simulink model "powerwindow_ec"  (R2019a)
settings: Solver=FixedStepDiscrete  StartTime=0.0  StopTime=20.0  FixedStep=0.01  RelTol=1e-3
values from neighbouring files (symbols this model uses):
  auto_down_time = copy(auto_up_time)    [powerwindow_ec_init.m]
  auto_up_time = Simulink.Parameter    [powerwindow_ec_init.m]
  bFALSE = Simulink.Parameter    [powerwindow_ec_init.m]
  emergency_down_time = copy(auto_up_time)    [powerwindow_ec_init.m]
  position_endstop_top = Simulink.Parameter    [powerwindow_ec_init.m]
settings Model: TunableVars=auto_down_time,auto_up_time,emergency_down_time,position_endstop_top  TunableVarsStorageClass=Auto,Auto,Auto,Auto  TunableVarsTypeQualifier=,,,  Creator=Wolfgang Meincke  LastModifiedBy=yatishc
settings DataIOCC: LimitDataPoints=on  SaveFormat=Array  ReturnWorkspaceOutputs=off
settings OptimizationCC: BlockReduction=off  BooleanDataType=off  ConditionallyExecuteInputs=off  DefaultParameterBehavior=Inlined  GlobalBufferReuse=off  EnableMemcpy=off  ExpressionDepthLimit=2147483647  ZeroExternalMemoryAtStartup=off  ZeroInternalMemoryAtStartup=off  InitFltsAndDblsToZero=on  NoFixptDivByZeroProtection=on  LifeSpan=1
settings DebuggingCC: RTPrefix=none  SaveWithParameterizedLinksMsg=none  UnderspecifiedInitializationDetection=Classic  MergeDetectMultiDrivingBlocksExec=none  MultiTaskDSMMsg=warning  MultiTaskCondExecSysMsg=none  ParameterPrecisionLossMsg=none  FcnCallInpInsideContextMsg=warning  UnconnectedInputMsg=none  UnconnectedOutputMsg=none  AllowSymbolicDim=off  StateNameClashWarn=warning  SFUnexpectedBacktrackingDiag=warning  SFNoUnconditionalDefaultTransitionDiag=warning  SFExecutionAtInitializationDiag=none  ArithmeticOperatorsInVariantConditions=warning
settings HardwareCC: ProdLongLongMode=on
settings ModelReferenceCC: ModelReferenceNumInstancesAllowed=Single  PropagateSignalLabelsOutOfModel=off
settings SFSimCC: SimUseLocalCustomCode=off  SimParseCustomCode=off  MATLABDynamicMemAlloc=off
settings RTWCC: SystemTargetFile=ert.tlc  GenCodeOnly=on  TemplateMakefile=ert_default_tmf  RetainRTWFile=on  RTWUseLocalCustomCode=off  Toolchain=LCC-win64 v2.4.1 | gmake (64-bit Windows)  PortableWordSizes=on
settings CodeAppCC: IgnoreCustomStorageClasses=off  MaxIdLength=40  StateflowObjectComments=on
settings ERTTargetCC: MultiwordLength=2048  IncludeMdlTerminateFcn=off  CombineSignalStateStructs=on  SupportAbsoluteTime=off  LogVarNameModifier=_rt  PurelyIntegerCode=on  SupportNonFinite=off  SupportComplex=off  RemoveResetFunc=off  RootIOFormat=Part of model data structure  ERTCustomFileTemplate=example_file_process.tlc  ConvertIfToSwitch=off  SuppressUnreachableDefaultCases=off
settings ConfigComp: CovMetricSettings=dw  CovSaveCumulativeToWorkspaceVar=on  CovSaveSingleToWorkspaceVar=on  CovExternalEMLEnable=off  CovSFcnEnable=off

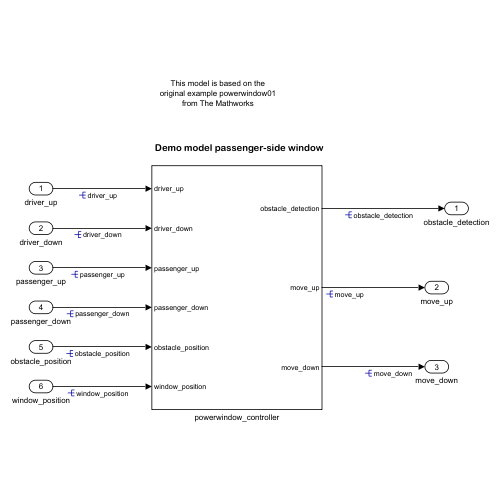
[thumbnail: Simulink's stored preview of the top-level diagram]
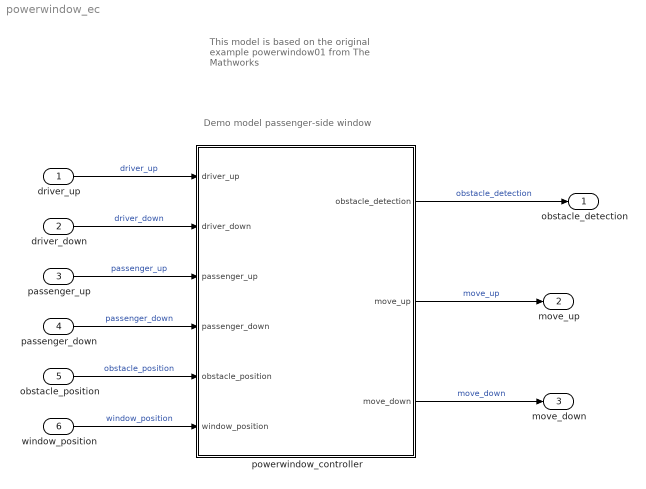
== system powerwindow_ec ==
  note: This model is based on the
      | original example powerwindow01
      | from The Mathworks
  note: Demo model passenger-side window
  driver_up : Inport  OutMin=0  OutMax=1
  driver_down : Inport  Port=2  OutMin=0  OutMax=1
  passenger_up : Inport  Port=3  OutMin=0  OutMax=1
  passenger_down : Inport  Port=4  OutMin=0  OutMax=1
  obstacle_position : Inport  Port=5  OutMin=0  OutMax=0.45  OutDataTypeStr=fixdt(0,16,0.001,0)
  window_position : Inport  Port=6  OutMin=0  OutMax=0.45  OutDataTypeStr=fixdt(0,16,0.001,0)
  powerwindow_controller : Subsystem  RTWFcnName=powerwindow_controller
      settings: RTWSystemCode=Nonreusable function  RTWFcnNameOpts=User specified  RTWFileNameOpts=Use function name
  obstacle_detection : Outport  OutMin=0  OutMax=1  VectorParamsAs1DForOutWhenUnconnected=off
  move_up : Outport  Port=2  OutMin=0  OutMax=1  VectorParamsAs1DForOutWhenUnconnected=off
  move_down : Outport  Port=3  OutMin=0  OutMax=1  VectorParamsAs1DForOutWhenUnconnected=off
  wires:
  driver_up/1 -> powerwindow_controller/1(driver_up)  "driver_up"
  driver_down/1 -> powerwindow_controller/2(driver_down)  "driver_down"
  passenger_up/1 -> powerwindow_controller/3(passenger_up)  "passenger_up"
  passenger_down/1 -> powerwindow_controller/4(passenger_down)  "passenger_down"
  obstacle_position/1 -> powerwindow_controller/5(obstacle_position)  "obstacle_position"
  window_position/1 -> powerwindow_controller/6(window_position)  "window_position"
  powerwindow_controller/1(obstacle_detection) -> obstacle_detection/1  "obstacle_detection"
  powerwindow_controller/2(move_up) -> move_up/1  "move_up"
  powerwindow_controller/3(move_down) -> move_down/1  "move_down"

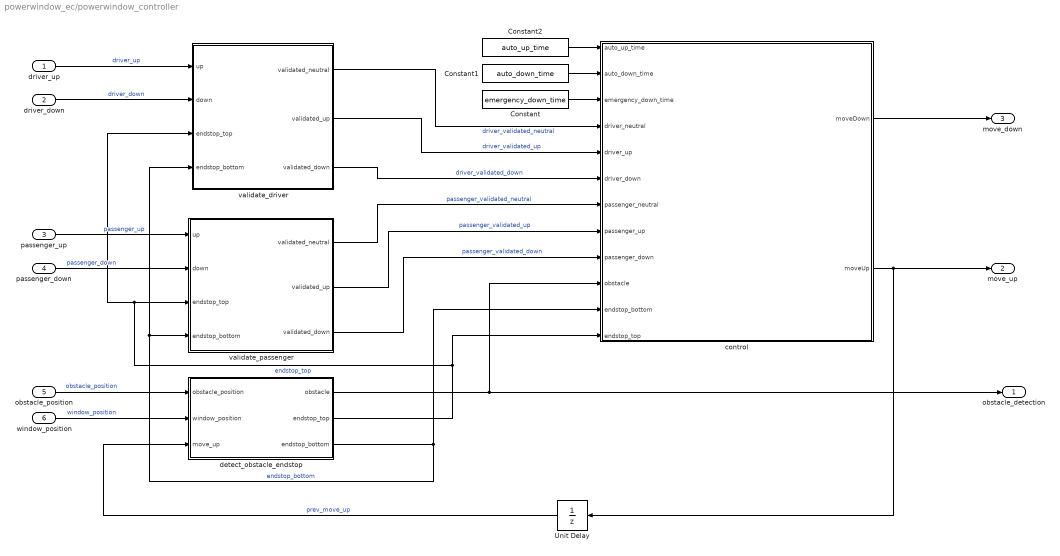
== system powerwindow_ec/powerwindow_controller ==
  driver_up : Inport  RequirementInfo={} %GIDa_c35cf34b_45f5_487d_8434_6977e2d5d2f3  OutMin=0  OutMax=1  OutDataTypeStr=boolean  PortDimensions=1
  driver_down : Inport  RequirementInfo={} %GIDa_825829a4_4c67_4036_abe4_d775b7ffbdb6  Port=2  OutMin=0  OutMax=1  OutDataTypeStr=boolean
  passenger_up : Inport  RequirementInfo={} %GIDa_896a61d0_51a5_427e_b548_01888eb9493f  Port=3  OutMin=0  OutMax=1  OutDataTypeStr=boolean  PortDimensions=1
  passenger_down : Inport  RequirementInfo={} %GIDa_acad868a_9832_4517_80f1_eb2c424aca82  Port=4  OutMin=0  OutMax=1  OutDataTypeStr=boolean  PortDimensions=1
  obstacle_position : Inport  RequirementInfo={} %GIDa_5be180b3_640c_44df_b132_7c12c9dd4782  Port=5  OutMin=0  OutMax=0.45  OutDataTypeStr=fixdt(0,16,0.001,0)  PortDimensions=1
  window_position : Inport  RequirementInfo={} %GIDa_279514cf_fecf_4861_97d0_86738c273b33  Port=6  OutMin=0  OutMax=0.45  OutDataTypeStr=fixdt(0,16,0.001,0)  PortDimensions=1
  Constant : Constant  RequirementInfo={} %GIDa_9514aab4_7290_4656_a952_a9cac9bec120  Value=emergency_down_time  OutMin=0  OutMax=255  OutDataTypeStr=uint8
  Constant1 : Constant  RequirementInfo={} %GIDa_6c74b792_e839_4a12_ac84_86c7d570a533  Value=auto_down_time  OutMin=0  OutMax=255  OutDataTypeStr=uint8
  Constant2 : Constant  RequirementInfo={} %GIDa_27bbea0c_c5f9_4e52_b093_a1cd3ec1797f  Value=auto_up_time  OutMin=0  OutMax=255  OutDataTypeStr=uint8
  Unit Delay : UnitDelay  RequirementInfo={} %GIDa_61c3f994_badd_4b85_b577_84166d45c76a  SampleTime=-1  HasFrameUpgradeWarning=on
  control : Stateflow chart  RequirementInfo={} %GIDa_03dc6751_b1fa_4801_9ce5_d6a4ecb5c081
      settings: FunctionInterfaceSpec=Allow arguments
  detect_obstacle_endstop : Subsystem  Description=""  TreatAsAtomicUnit=on  RTWFcnName=detect_obstacle_endstop
      settings: AttributesFormatString=%<Description>  RTWSystemCode=Nonreusable function  RTWFcnNameOpts=User specified  RTWFileNameOpts=Use subsystem name
  validate_driver : Subsystem  TreatAsAtomicUnit=on  RTWFcnName=validate_driver
      settings: RTWSystemCode=Nonreusable function  RTWFcnNameOpts=User specified  RTWFileNameOpts=Use subsystem name
  validate_passenger : Subsystem  RequirementInfo={} %GIDa_33b218b3_9db5_4fe6_9638_6b05429d8e58  TreatAsAtomicUnit=on  RTWFcnName=validate_passenger
      settings: RTWSystemCode=Nonreusable function  RTWFcnNameOpts=User specified  RTWFileNameOpts=Use function name
  obstacle_detection : Outport  RequirementInfo={} %GIDa_4eefd6fd_6a0d_4232_ac82_ccb47f3c36e3  OutMin=0  OutMax=1  OutDataTypeStr=boolean  PortDimensions=1  VectorParamsAs1DForOutWhenUnconnected=off
  move_up : Outport  RequirementInfo={} %GIDa_cfaa6890_1b09_43c8_9181_c9775bd2e746  Port=2  OutMin=0  OutMax=1  OutDataTypeStr=boolean  PortDimensions=1  VectorParamsAs1DForOutWhenUnconnected=off
  move_down : Outport  RequirementInfo={} %GIDa_e72b7e0a_8232_4793_901f_580fad4f0530  Port=3  OutMin=0  OutMax=1  OutDataTypeStr=boolean  PortDimensions=1  VectorParamsAs1DForOutWhenUnconnected=off
  wires:
  detect_obstacle_endstop/3(endstop_bottom) -> validate_driver/4(endstop_bottom), validate_passenger/4(endstop_bottom), control/11(endstop_bottom)  "endstop_bottom"
  detect_obstacle_endstop/2(endstop_top) -> control/12(endstop_top), validate_driver/3(endstop_top), validate_passenger/3(endstop_top)  "endstop_top"
  validate_passenger/3(validated_down) -> control/9(passenger_down)  "passenger_validated_down"
  validate_passenger/2(validated_up) -> control/8(passenger_up)  "passenger_validated_up"
  validate_passenger/1(validated_neutral) -> control/7(passenger_neutral)  "passenger_validated_neutral"
  validate_driver/3(validated_down) -> control/6(driver_down)  "driver_validated_down"
  validate_driver/2(validated_up) -> control/5(driver_up)  "driver_validated_up"
  validate_driver/1(validated_neutral) -> control/4(driver_neutral)  "driver_validated_neutral"
  Constant/1 -> control/3(emergency_down_time)
  Constant1/1 -> control/2(auto_down_time)
  Constant2/1 -> control/1(auto_up_time)
  control/1(moveDown) -> move_down/1
  control/2(moveUp) -> move_up/1, Unit Delay/1
  detect_obstacle_endstop/1(obstacle) -> control/10(obstacle), obstacle_detection/1
  Unit Delay/1 -> detect_obstacle_endstop/3(move_up)  "prev_move_up"
  window_position/1 -> detect_obstacle_endstop/2(window_position)  "window_position"
  obstacle_position/1 -> detect_obstacle_endstop/1(obstacle_position)  "obstacle_position"
  passenger_down/1 -> validate_passenger/2(down)  "passenger_down"
  passenger_up/1 -> validate_passenger/1(up)  "passenger_up"
  driver_down/1 -> validate_driver/2(down)  "driver_down"
  driver_up/1 -> validate_driver/1(up)  "driver_up"

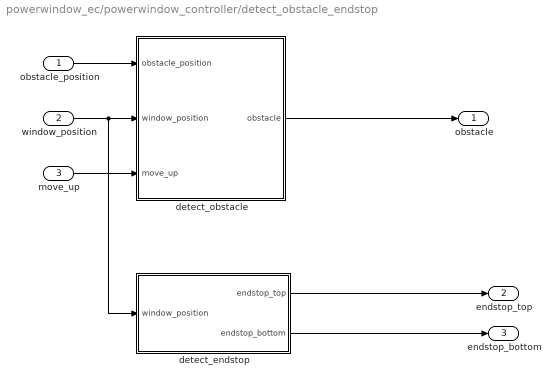
== system powerwindow_ec/powerwindow_controller/detect_obstacle_endstop ==
  obstacle_position : Inport  RequirementInfo={} %GIDa_2c523ff6_7978_4731_916d_ba96442347ee
  window_position : Inport  RequirementInfo={} %GIDa_e1d20317_e3ef_4a09_9a0f_4281293c9f26  Port=2
  move_up : Inport  RequirementInfo={} %GIDa_5f38f6b1_95fb_4aef_ba44_8aaabe685aa5  Port=3
  detect_endstop : Subsystem  RequirementInfo={} %GIDa_2593335f_ebb0_43cf_9a39_2217339a862c
  detect_obstacle : Subsystem  RequirementInfo={} %GIDa_68f09a5d_865e_4d80_9553_6123df56ce2c
  obstacle : Outport  RequirementInfo={} %GIDa_76b93d49_6133_4f74_9957_e79afe91ce74  VectorParamsAs1DForOutWhenUnconnected=off
  endstop_top : Outport  RequirementInfo={} %GIDa_88a654a8_9697_4d16_b6ed_e9fe94316691  Port=2  VectorParamsAs1DForOutWhenUnconnected=off
  endstop_bottom : Outport  RequirementInfo={} %GIDa_79e1bc3d_40d8_4ea1_ab03_899f1380a234  Port=3  VectorParamsAs1DForOutWhenUnconnected=off
  wires:
  detect_endstop/2(endstop_bottom) -> endstop_bottom/1
  detect_endstop/1(endstop_top) -> endstop_top/1
  detect_obstacle/1(obstacle) -> obstacle/1
  obstacle_position/1 -> detect_obstacle/1(obstacle_position)
  window_position/1 -> detect_endstop/1(window_position), detect_obstacle/2(window_position)
  move_up/1 -> detect_obstacle/3(move_up)

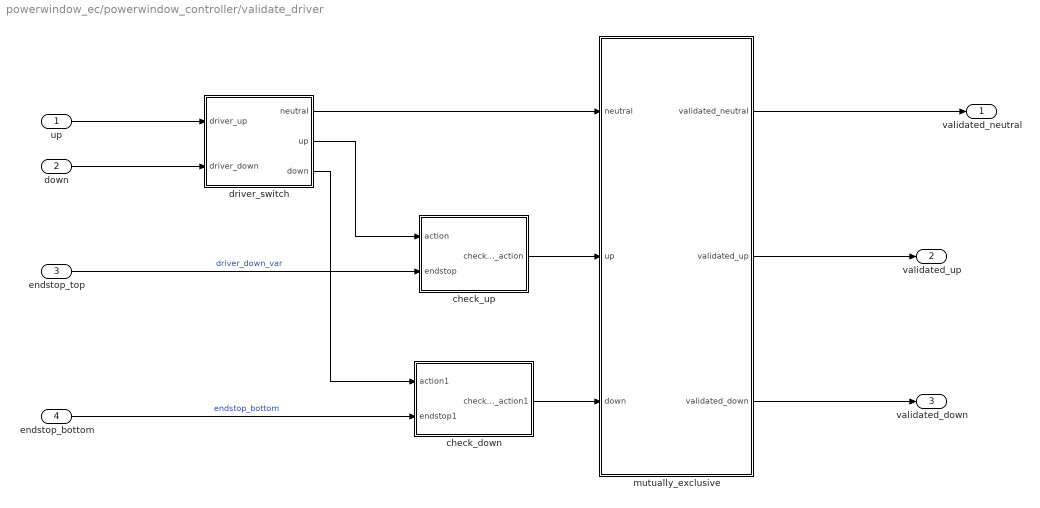
== system powerwindow_ec/powerwindow_controller/validate_driver ==
  up : Inport  RequirementInfo={} %GIDa_0f060a46_f46d_4ca9_9fdd_5b4ef64425ee  OutDataTypeStr=boolean  PortDimensions=1  SampleTime=[0.01,0]
  down : Inport  RequirementInfo={} %GIDa_ee71ce1a_69e4_43ae_938d_beeecc753a79  Port=2  OutDataTypeStr=boolean  PortDimensions=1  SampleTime=[0.01,0]
  endstop_top : Inport  RequirementInfo={} %GIDa_950bdb33_ed63_463b_ae82_db42f04fc79f  Port=3  OutDataTypeStr=boolean  PortDimensions=1  SampleTime=[0.01,0]
  endstop_bottom : Inport  RequirementInfo={} %GIDa_82fa3d1b_deb6_4fcf_98df_c73a1f0760dd  Port=4  OutDataTypeStr=boolean  PortDimensions=1  SampleTime=[0.01,0]
  check_down : Subsystem  RequirementInfo={} %GIDa_88cdc8aa_9e17_4d6d_82ad_f4b053a158b5
  check_up : Subsystem  RequirementInfo={} %GIDa_f004a38e_b1e3_4775_9b61_543b39059229
  driver_switch : Subsystem  RequirementInfo={} %GIDa_0ddca807_3145_43f8_91cf_ba07f3905be6
  mutually_exclusive : Subsystem  RequirementInfo={} %GIDa_48603077_07ff_4607_938a_0c2458af8a7a
  validated_neutral : Outport  RequirementInfo={} %GIDa_93510d49_6043_4ebc_8207_b7ce98567d3f  OutDataTypeStr=boolean  PortDimensions=1  SampleTime=[0.01,0]  VectorParamsAs1DForOutWhenUnconnected=off
  validated_up : Outport  RequirementInfo={} %GIDa_e717bde8_9582_4b32_98f4_cb8fdf2291d3  Port=2  OutDataTypeStr=boolean  PortDimensions=1  SampleTime=[0.01,0]  VectorParamsAs1DForOutWhenUnconnected=off
  validated_down : Outport  RequirementInfo={} %GIDa_99f1727e_ebb0_4d17_9343_1d6808b3939a  Port=3  OutDataTypeStr=boolean  PortDimensions=1  SampleTime=[0.01,0]  VectorParamsAs1DForOutWhenUnconnected=off
  wires:
  mutually_exclusive/3(validated_down) -> validated_down/1
  mutually_exclusive/2(validated_up) -> validated_up/1
  mutually_exclusive/1(validated_neutral) -> validated_neutral/1
  check_down/1(checked_action1) -> mutually_exclusive/3(down)
  check_up/1(checked_action) -> mutually_exclusive/2(up)
  driver_switch/1(neutral) -> mutually_exclusive/1(neutral)
  endstop_bottom/1 -> check_down/2(endstop1)  "endstop_bottom"
  endstop_top/1 -> check_up/2(endstop)  "driver_down_var"
  driver_switch/3(down) -> check_down/1(action1)
  driver_switch/2(up) -> check_up/1(action)
  down/1 -> driver_switch/2(driver_down)
  up/1 -> driver_switch/1(driver_up)

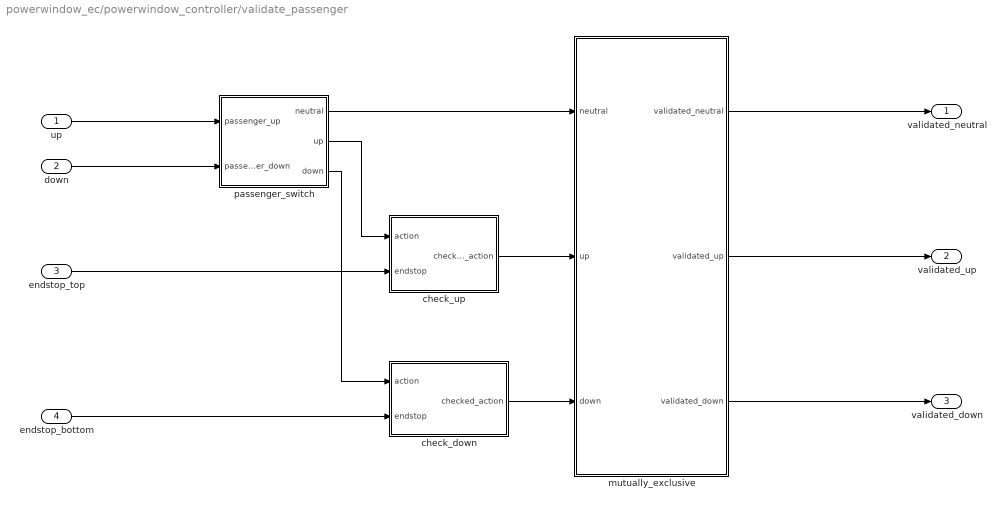
== system powerwindow_ec/powerwindow_controller/validate_passenger ==
  up : Inport  RequirementInfo={} %GIDa_b6408152_b334_4925_a16c_3622ca90ad97
  down : Inport  RequirementInfo={} %GIDa_df58e8e8_afe3_46fe_9c17_76802ca163b9  Port=2
  endstop_top : Inport  RequirementInfo={} %GIDa_230b0d07_e7b6_4a10_b2ed_43443fa38605  Port=3
  endstop_bottom : Inport  RequirementInfo={} %GIDa_91eacfdf_7e8f_4c54_b206_f15636a3f59e  Port=4
  check_down : Subsystem  RequirementInfo={} %GIDa_62b405b0_f053_4287_a6d2_c18d3e3b6c5b
  check_up : Subsystem  RequirementInfo={} %GIDa_92e78854_fa4d_4c59_81d3_3ea0d0c4a8a4
  mutually_exclusive : Subsystem  RequirementInfo={} %GIDa_5d841e18_2fc4_47d2_8782_e39db535edd2
  passenger_switch : Subsystem  RequirementInfo={} %GIDa_1746543f_6789_44d7_a576_254e44230f82
  validated_neutral : Outport  RequirementInfo={} %GIDa_ebd107f4_f924_4fcc_86d4_5bdc2b7613d2  VectorParamsAs1DForOutWhenUnconnected=off
  validated_up : Outport  RequirementInfo={} %GIDa_a655668a_fb1a_4125_a470_9ec06e9de417  Port=2  VectorParamsAs1DForOutWhenUnconnected=off
  validated_down : Outport  RequirementInfo={} %GIDa_d891aac2_9896_4b15_add3_213d9f963ba8  Port=3  VectorParamsAs1DForOutWhenUnconnected=off
  wires:
  check_down/1(checked_action) -> mutually_exclusive/3(down)
  check_up/1(checked_action) -> mutually_exclusive/2(up)
  passenger_switch/1(neutral) -> mutually_exclusive/1(neutral)
  endstop_bottom/1 -> check_down/2(endstop)
  endstop_top/1 -> check_up/2(endstop)
  passenger_switch/3(down) -> check_down/1(action)
  passenger_switch/2(up) -> check_up/1(action)
  down/1 -> passenger_switch/2(passenger_down)
  up/1 -> passenger_switch/1(passenger_up)
  mutually_exclusive/1(validated_neutral) -> validated_neutral/1
  mutually_exclusive/2(validated_up) -> validated_up/1
  mutually_exclusive/3(validated_down) -> validated_down/1

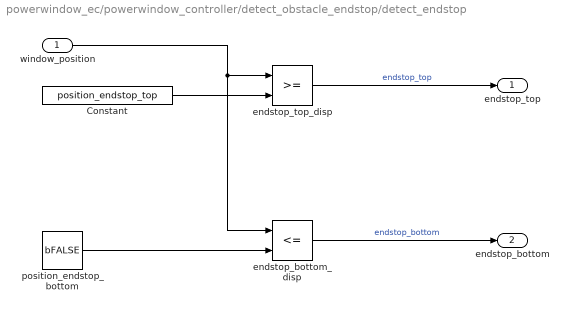
== system powerwindow_ec/powerwindow_controller/detect_obstacle_endstop/detect_endstop ==
  window_position : Inport  RequirementInfo={} %GIDa_5272641f_60a5_49ab_860f_474d665ad38c
  Constant : Constant  RequirementInfo={} %GIDa_b00b9cbe_3e72_4b2c_8740_e9f730c36594  Value=position_endstop_top  OutMin=0.35  OutMax=0.45  OutDataTypeStr=fixdt(0,16,0.001,0)
  endstop_bottom_disp : RelationalOperator  RequirementInfo={} %GIDa_d55d2907_c327_453e_a02b_45678f8411a7  Operator=<=  OutDataTypeStr=boolean  RndMeth=Nearest
      settings: AttributesFormatString=%<Description>
  endstop_top_disp : RelationalOperator  RequirementInfo={} %GIDa_6f4ae952_2810_4851_a41e_34cbed529beb  OutDataTypeStr=boolean  RndMeth=Nearest
      settings: AttributesFormatString=%<Description>
  position_endstop_bottom : Constant  RequirementInfo={} %GIDa_07897626_90bb_46f7_9dcd_03d3ee392bc4  Value=bFALSE  OutDataTypeStr=Inherit: Inherit via back propagation
  endstop_top : Outport  RequirementInfo={} %GIDa_6bdb3a67_ce18_47c7_a161_80224aafb80a  VectorParamsAs1DForOutWhenUnconnected=off
  endstop_bottom : Outport  RequirementInfo={} %GIDa_4cae9334_ebd9_4f06_b7b7_b5123c42f3a3  Port=2  VectorParamsAs1DForOutWhenUnconnected=off
  wires:
  endstop_bottom_disp/1 -> endstop_bottom/1  "endstop_bottom"
  endstop_top_disp/1 -> endstop_top/1  "endstop_top"
  position_endstop_bottom/1 -> endstop_bottom_disp/2
  window_position/1 -> endstop_bottom_disp/1, endstop_top_disp/1
  Constant/1 -> endstop_top_disp/2

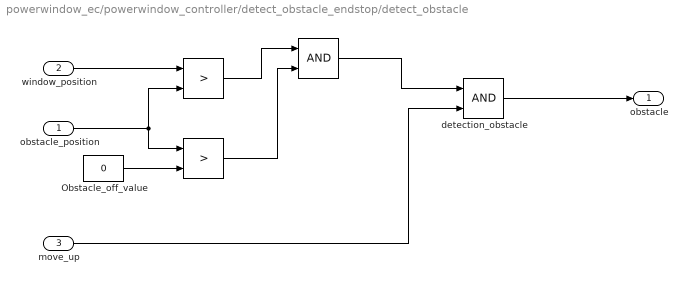
== system powerwindow_ec/powerwindow_controller/detect_obstacle_endstop/detect_obstacle ==
  obstacle_position : Inport  RequirementInfo={} %GIDa_f04cc014_84fe_4f3b_ba9a_4eb089b94b63
  window_position : Inport  RequirementInfo={} %GIDa_6efc2069_33c6_4baf_bb03_5d2172fe3169  Port=2
  move_up : Inport  RequirementInfo={} %GIDa_bfb3c774_9ca6_457c_ba9e_d7bb12997122  Port=3
  " " : Logic  RequirementInfo={} %GIDa_42f9d249_5a3b_49ec_af0d_2273563bb9a1  AllPortsSameDT=off  OutDataTypeStr=boolean
  "  " : RelationalOperator  RequirementInfo={} %GIDa_343b1761_e03d_4050_a63c_743fa9e53550  Operator=>  OutDataTypeStr=boolean  RndMeth=Nearest
  "   " : RelationalOperator  RequirementInfo={} %GIDa_d6c6c9bb_2e51_4c9f_94b3_dde6a683bc5b  Operator=>  OutDataTypeStr=boolean  RndMeth=Nearest
  Obstacle_off_value : Constant  RequirementInfo={} %GIDa_540ff0bd_b260_4aef_ac1e_5afd8b8de081  Value=0  OutDataTypeStr=Inherit: Inherit via back propagation
  detection_obstacle : Logic  RequirementInfo={} %GIDa_5a6fd671_9493_4039_aef6_1fac1883fec8  AllPortsSameDT=off  OutDataTypeStr=boolean
      settings: AttributesFormatString=%<Description>
  obstacle : Outport  RequirementInfo={} %GIDa_ab82724c_4453_4aa5_ac53_ecd73d5c0fd6  VectorParamsAs1DForOutWhenUnconnected=off
  wires:
  Obstacle_off_value/1 -> "   "/2
  obstacle_position/1 -> "  "/2, "   "/1
  "   "/1 -> " "/2
  move_up/1 -> detection_obstacle/2
  " "/1 -> detection_obstacle/1
  "  "/1 -> " "/1
  window_position/1 -> "  "/1
  detection_obstacle/1 -> obstacle/1

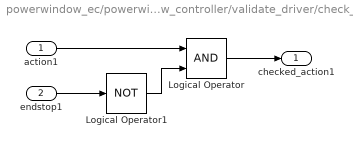
== system powerwindow_ec/powerwindow_controller/validate_driver/check_down ==
  action1 : Inport  RequirementInfo={} %GIDa_3bea607a_e8f1_4bd2_a5f0_c2e6970bbc31
  endstop1 : Inport  RequirementInfo={} %GIDa_b30aff22_abef_418a_aed3_192febbd33c5  Port=2
  Logical Operator : Logic  AllPortsSameDT=off  OutDataTypeStr=boolean
  Logical Operator1 : Logic  Operator=NOT  Inputs=1  AllPortsSameDT=off  OutDataTypeStr=boolean
  checked_action1 : Outport  RequirementInfo={} %GIDa_8daec588_ef56_4936_8f9d_ed4af0951a10  VectorParamsAs1DForOutWhenUnconnected=off
  wires:
  endstop1/1 -> Logical Operator1/1
  Logical Operator/1 -> checked_action1/1
  Logical Operator1/1 -> Logical Operator/2
  action1/1 -> Logical Operator/1

== system powerwindow_ec/powerwindow_controller/validate_driver/check_up ==
  action : Inport  RequirementInfo={} %GIDa_9887e9dd_28c6_4b8e_b0fa_e095af16b520
  endstop : Inport  RequirementInfo={} %GIDa_79f905fe_3050_4c1a_8e5e_85f3f37208eb  Port=2
  allow_action : Logic  RequirementInfo={} %GIDa_09215300_f454_41b9_9b13_3a6b54dcdb01  AllPortsSameDT=off  OutDataTypeStr=boolean
  not : Logic  RequirementInfo={} %GIDa_be8a7272_98c5_4194_9012_a918274462da  Operator=NOT  Inputs=1  AllPortsSameDT=off  OutDataTypeStr=boolean
  checked_action : Outport  RequirementInfo={} %GIDa_b7f1b7cb_7832_4f29_af81_202507dbc915  VectorParamsAs1DForOutWhenUnconnected=off
  wires:
  allow_action/1 -> checked_action/1  "checked_action"
  action/1 -> allow_action/1
  endstop/1 -> not/1
  not/1 -> allow_action/2

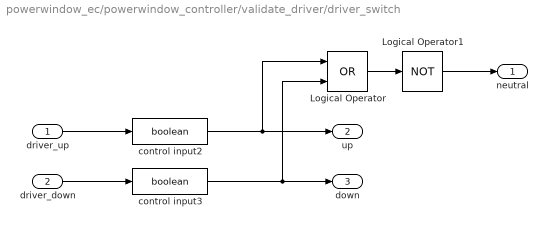
== system powerwindow_ec/powerwindow_controller/validate_driver/driver_switch ==
  driver_up : Inport  RequirementInfo={} %GIDa_b53eff7b_7dc7_4b26_a194_aca0440f3996
  driver_down : Inport  RequirementInfo={} %GIDa_850956fa_c58b_4722_af1c_699108fc9784  Port=2
  Logical Operator : Logic  RequirementInfo={} %GIDa_8ae19579_a7a5_4eb8_a8aa_b68c217ba182  Operator=OR  AllPortsSameDT=off  OutDataTypeStr=boolean
  Logical Operator1 : Logic  RequirementInfo={} %GIDa_e8e7857d_ce8d_43ef_928a_5ed594e12653  Operator=NOT  Inputs=1  AllPortsSameDT=off  OutDataTypeStr=boolean
  control input2 : DataTypeConversion  RequirementInfo={} %GIDa_c304843a_b249_46a1_bea1_8ad250524def  OutDataTypeStr=boolean  SaturateOnIntegerOverflow=on  RndMeth=Zero
  control input3 : DataTypeConversion  RequirementInfo={} %GIDa_1c10a33f_0b47_4b11_a97c_aa2c91a9423b  OutDataTypeStr=boolean  SaturateOnIntegerOverflow=on  RndMeth=Zero
  neutral : Outport  RequirementInfo={} %GIDa_6e66f8dd_3723_444f_a5c4_c8719978f12f  VectorParamsAs1DForOutWhenUnconnected=off
  up : Outport  RequirementInfo={} %GIDa_05276151_0839_48b1_ac06_cf6d99189f1e  Port=2  VectorParamsAs1DForOutWhenUnconnected=off
  down : Outport  RequirementInfo={} %GIDa_0ba51152_1781_4604_a294_81c93cdb2e1b  Port=3  VectorParamsAs1DForOutWhenUnconnected=off
  wires:
  driver_up/1 -> control input2/1
  driver_down/1 -> control input3/1
  control input2/1 -> up/1, Logical Operator/1
  control input3/1 -> down/1, Logical Operator/2
  Logical Operator/1 -> Logical Operator1/1
  Logical Operator1/1 -> neutral/1

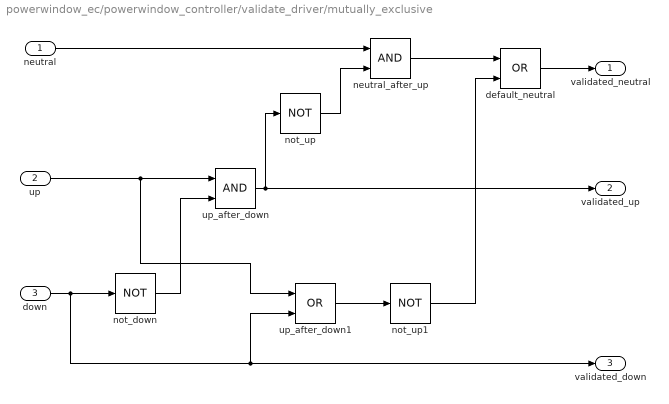
== system powerwindow_ec/powerwindow_controller/validate_driver/mutually_exclusive ==
  neutral : Inport  RequirementInfo={} %GIDa_02afa0c6_3e9f_4860_8ea3_38f0b34e8af7
  up : Inport  RequirementInfo={} %GIDa_1ebb9c89_44c5_40ac_900f_75ef026c92ad  Port=2
  down : Inport  RequirementInfo={} %GIDa_ad4b4981_c47d_4d30_8d96_b337e2a28fab  Port=3
  default_neutral : Logic  RequirementInfo={} %GIDa_68c2c660_39d6_4c62_9a3a_19199413336b  Operator=OR  AllPortsSameDT=off  OutDataTypeStr=boolean
  neutral_after_up : Logic  RequirementInfo={} %GIDa_7e258c9e_2c01_4723_a13f_4f5e92480034  AllPortsSameDT=off  OutDataTypeStr=boolean
  not_down : Logic  RequirementInfo={} %GIDa_a256d950_ec2d_4e87_a052_2312a72abf35  Operator=NOT  Inputs=1  AllPortsSameDT=off  OutDataTypeStr=boolean
  not_up : Logic  RequirementInfo={} %GIDa_f2e45f11_593e_44a0_9f62_a4dedafdeaaa  Operator=NOT  Inputs=1  AllPortsSameDT=off  OutDataTypeStr=boolean
  not_up1 : Logic  RequirementInfo={} %GIDa_57241b58_9572_4fb8_96d3_b88159c194b1  Operator=NOT  Inputs=1  AllPortsSameDT=off  OutDataTypeStr=boolean
  up_after_down : Logic  RequirementInfo={} %GIDa_f2858def_6366_414f_b896_53e3e935ca29  AllPortsSameDT=off  OutDataTypeStr=boolean
  up_after_down1 : Logic  RequirementInfo={} %GIDa_c5cf92de_e71e_48a0_b3a2_b9222e289e08  Operator=OR  AllPortsSameDT=off  OutDataTypeStr=boolean
  validated_neutral : Outport  RequirementInfo={} %GIDa_5fe76ab9_064b_4710_a12f_97d13d073964  VectorParamsAs1DForOutWhenUnconnected=off
  validated_up : Outport  RequirementInfo={} %GIDa_2868f914_1275_4356_93d2_c378fc22247d  Port=2  VectorParamsAs1DForOutWhenUnconnected=off
  validated_down : Outport  RequirementInfo={} %GIDa_b1de4b41_5c80_4a3b_8187_9415b836eb74  Port=3  VectorParamsAs1DForOutWhenUnconnected=off
  wires:
  neutral/1 -> neutral_after_up/1
  not_up/1 -> neutral_after_up/2
  up_after_down/1 -> validated_up/1, not_up/1
  up/1 -> up_after_down/1, up_after_down1/1
  down/1 -> not_down/1, validated_down/1, up_after_down1/2
  not_down/1 -> up_after_down/2
  up_after_down1/1 -> not_up1/1
  not_up1/1 -> default_neutral/2
  neutral_after_up/1 -> default_neutral/1
  default_neutral/1 -> validated_neutral/1

== system powerwindow_ec/powerwindow_controller/validate_passenger/check_down ==
  action : Inport  RequirementInfo={} %GIDa_ca512674_cbe4_48ba_9017_69e0f816f711
  endstop : Inport  RequirementInfo={} %GIDa_59664dfc_9454_41cf_927b_a889b06514c8  Port=2
  allow_action : Logic  RequirementInfo={} %GIDa_6d61b7cc_cf4f_459c_8f84_8bb0cf779dee  AllPortsSameDT=off  OutDataTypeStr=boolean
  not : Logic  RequirementInfo={} %GIDa_75feb0d0_87dd_4abc_903e_36f510d82096  Operator=NOT  Inputs=1  AllPortsSameDT=off  OutDataTypeStr=boolean
  checked_action : Outport  RequirementInfo={} %GIDa_6a46bd9b_176e_4e3e_a6a8_fff5e40471e2  VectorParamsAs1DForOutWhenUnconnected=off
  wires:
  action/1 -> allow_action/1
  not/1 -> allow_action/2
  allow_action/1 -> checked_action/1  "checked_action"
  endstop/1 -> not/1

== system powerwindow_ec/powerwindow_controller/validate_passenger/check_up ==
  action : Inport  RequirementInfo={} %GIDa_dc7fa4e4_fe57_40ae_a062_8dffeb9176be
  endstop : Inport  RequirementInfo={} %GIDa_5af3944e_bdc7_478a_9674_1af1981846f4  Port=2
  allow_action : Logic  RequirementInfo={} %GIDa_96999e18_96cd_470f_ae60_b66afebaee89  AllPortsSameDT=off  OutDataTypeStr=boolean
  not : Logic  RequirementInfo={} %GIDa_a0499630_f6e4_41e6_ae99_6236f2ab45db  Operator=NOT  Inputs=1  AllPortsSameDT=off  OutDataTypeStr=boolean
  checked_action : Outport  RequirementInfo={} %GIDa_8039e34e_7a32_4eab_98be_7588d21475d6  VectorParamsAs1DForOutWhenUnconnected=off
  wires:
  not/1 -> allow_action/2
  endstop/1 -> not/1
  action/1 -> allow_action/1
  allow_action/1 -> checked_action/1  "checked_action"

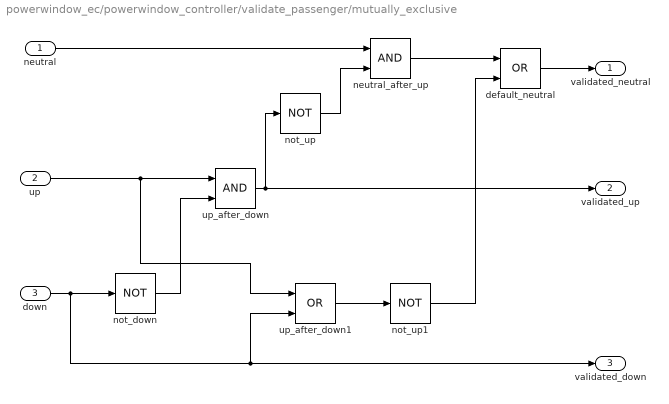
== system powerwindow_ec/powerwindow_controller/validate_passenger/mutually_exclusive ==
  neutral : Inport  RequirementInfo={} %GIDa_8f003c53_0f06_402c_bf11_e1dae5ac4ba2
  up : Inport  RequirementInfo={} %GIDa_13e7cfed_65e8_4439_989f_1cf26328e825  Port=2
  down : Inport  RequirementInfo={} %GIDa_b18b33e4_0100_4836_9df2_c076b889bc83  Port=3
  default_neutral : Logic  RequirementInfo={} %GIDa_721e8f87_b194_487a_970a_3a929a776efa  Operator=OR  AllPortsSameDT=off  OutDataTypeStr=boolean
  neutral_after_up : Logic  RequirementInfo={} %GIDa_099c4db0_1ced_407c_9a11_52cdc433151a  AllPortsSameDT=off  OutDataTypeStr=boolean
  not_down : Logic  RequirementInfo={} %GIDa_21e7df57_4079_420c_aa24_638c8886d47b  Operator=NOT  Inputs=1  AllPortsSameDT=off  OutDataTypeStr=boolean
  not_up : Logic  RequirementInfo={} %GIDa_ba891d16_2ab0_4455_8efb_8452a25ddce4  Operator=NOT  Inputs=1  AllPortsSameDT=off  OutDataTypeStr=boolean
  not_up1 : Logic  RequirementInfo={} %GIDa_d7755c1f_7020_4217_ac48_627cd233c0c5  Operator=NOT  Inputs=1  AllPortsSameDT=off  OutDataTypeStr=boolean
  up_after_down : Logic  RequirementInfo={} %GIDa_6c1a5302_81e3_4f31_8645_f01e65565135  AllPortsSameDT=off  OutDataTypeStr=boolean
  up_after_down1 : Logic  RequirementInfo={} %GIDa_68cb3128_3b52_420a_b6c5_4a84693a377b  Operator=OR  AllPortsSameDT=off  OutDataTypeStr=boolean
  validated_neutral : Outport  RequirementInfo={} %GIDa_49ff77a4_e54e_4e57_8264_91fcfa71c2f8  VectorParamsAs1DForOutWhenUnconnected=off
  validated_up : Outport  RequirementInfo={} %GIDa_c13404c1_0905_4a17_a186_e38525a7269f  Port=2  VectorParamsAs1DForOutWhenUnconnected=off
  validated_down : Outport  RequirementInfo={} %GIDa_f8e3c94c_9fee_405f_8ae0_09bb929cc26c  Port=3  VectorParamsAs1DForOutWhenUnconnected=off
  wires:
  default_neutral/1 -> validated_neutral/1
  neutral_after_up/1 -> default_neutral/1
  not_up1/1 -> default_neutral/2
  up_after_down1/1 -> not_up1/1
  not_down/1 -> up_after_down/2
  down/1 -> up_after_down1/2, validated_down/1, not_down/1
  up/1 -> up_after_down1/1, up_after_down/1
  up_after_down/1 -> not_up/1, validated_up/1
  not_up/1 -> neutral_after_up/2
  neutral/1 -> neutral_after_up/1

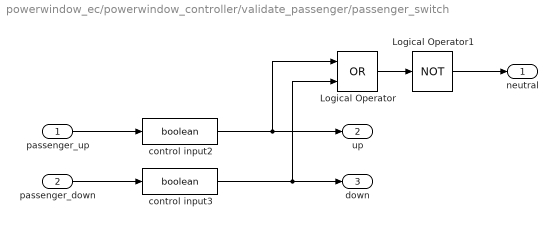
== system powerwindow_ec/powerwindow_controller/validate_passenger/passenger_switch ==
  passenger_up : Inport  RequirementInfo={} %GIDa_61b4d6eb_b343_41f6_8a80_dcc5328050d4
  passenger_down : Inport  RequirementInfo={} %GIDa_159ae53f_aacb_4aa9_ab9b_f7d3b5ed93b6  Port=2
  Logical Operator : Logic  RequirementInfo={} %GIDa_7d1f1e29_2525_49a5_8297_8d1857c67a70  Operator=OR  AllPortsSameDT=off  OutDataTypeStr=boolean
  Logical Operator1 : Logic  RequirementInfo={} %GIDa_c67391d6_db29_412d_911b_665d5b7f1999  Operator=NOT  Inputs=1  AllPortsSameDT=off  OutDataTypeStr=boolean
  control input2 : DataTypeConversion  RequirementInfo={} %GIDa_15e65c4a_7f2f_4a03_ad86_98d237be47e6  OutDataTypeStr=boolean  SaturateOnIntegerOverflow=on  RndMeth=Zero
  control input3 : DataTypeConversion  RequirementInfo={} %GIDa_44021398_892f_4942_b995_99cb371ef146  OutDataTypeStr=boolean  SaturateOnIntegerOverflow=on  RndMeth=Zero
  neutral : Outport  RequirementInfo={} %GIDa_82178efc_15f5_4b92_893f_50e480dd7654  VectorParamsAs1DForOutWhenUnconnected=off
  up : Outport  RequirementInfo={} %GIDa_9ba8bbc2_f4d4_4c2a_a343_4354814556d4  Port=2  VectorParamsAs1DForOutWhenUnconnected=off
  down : Outport  RequirementInfo={} %GIDa_e2954a87_897d_46fb_be12_5a148406f165  Port=3  VectorParamsAs1DForOutWhenUnconnected=off
  wires:
  Logical Operator1/1 -> neutral/1
  Logical Operator/1 -> Logical Operator1/1
  control input3/1 -> Logical Operator/2, down/1
  control input2/1 -> Logical Operator/1, up/1
  passenger_down/1 -> control input3/1
  passenger_up/1 -> control input2/1

== stateflow chart powerwindow_ec/powerwindow_controller/control ==
  state safe
    state driverNeutral
      entry:
      moveUp = 0;
      moveDown = 0;
      state passengerneutral
        entry:
        moveUp = 0;
        moveDown = 0;
      state passengerDown
        entry: moveDown = 1;
        exit:   moveDown = 0;
        state iniPassengerDown
        state passengerDown
        state autoPassengerDown
        iniPassengerDown -> (junction 14) : after(auto_down_time,tick)
        (junction 14) -> safe.driverNeutral.passengerDown.passengerDown [order 2]
        (junction 14) -> autoPassengerDown [order 1] : [passenger_neutral]
      state passengerUp
        entry: moveUp = 1;
        exit: moveUp = 0;
        state iniPassengerUp
        state PassengerUp
        state autoPassengerUp
        iniPassengerUp -> (junction 29) : after(auto_up_time,tick)
        (junction 29) -> PassengerUp [order 2]
        (junction 29) -> autoPassengerUp [order 1] : [passenger_neutral]
      (default) -> passengerneutral
      passengerneutral -> iniPassengerUp [order 1] : [passenger_up]
      passengerneutral -> iniPassengerDown [order 2] : [passenger_down]
      safe.driverNeutral.passengerDown.passengerDown -> passengerneutral : [passenger_neutral]
      PassengerUp -> passengerneutral : [passenger_neutral]
      safe.driverNeutral.passengerDown -> passengerneutral [order 1] : [endstop_bottom]
      passengerUp -> passengerneutral [order 2] : [endstop_top]
      safe.driverNeutral.passengerDown -> PassengerUp [order 2] : [passenger_up]
      passengerUp -> safe.driverNeutral.passengerDown.passengerDown [order 1] : [passenger_down]
    state driverUp
      entry: moveUp = 1;
      exit: moveUp = 0;
      state iniDriverUp
      state DriverUp
      state autoDriverUp
      iniDriverUp -> (junction 55) : after(auto_up_time,tick)
      (junction 55) -> DriverUp [order 2]
      (junction 55) -> autoDriverUp [order 1] : [driver_neutral]
    state driverDown
      entry: moveDown = 1;
      exit: moveDown = 0;
      state iniDriverDown
      state DriverDown
      state autoDriverDown
      iniDriverDown -> (junction 44) : after(auto_down_time,tick)
      (junction 44) -> DriverDown [order 2]
      (junction 44) -> autoDriverDown [order 1] : [driver_neutral]
    (default) -> driverNeutral
    driverNeutral -> iniDriverDown [order 2] : [driver_down]
    DriverDown -> driverNeutral : [driver_neutral]
    driverDown -> driverNeutral [order 1] : [endstop_bottom]
    DriverUp -> driverNeutral : [driver_neutral]
    driverUp -> driverNeutral [order 2] : [endstop_top]
    driverNeutral -> iniDriverUp [order 1] : [driver_up]
    driverDown -> DriverUp [order 2] : [driver_up]
    driverUp -> DriverDown [order 1] : [driver_down]
  state emergencyDown
    entry:
    moveUp = 0;
    moveDown = 1;
  emergencyDown -> passengerneutral : [endstop_bottom | after(emergency_down_time,tick)]
  (default) -> safe
  safe -> emergencyDown : [obstacle]
  data: auto_up_time input; auto_down_time input; emergency_down_time input; driver_neutral input; driver_up input; driver_down input; passenger_neutral input; passenger_up input; passenger_down input; obstacle input; endstop_bottom input; endstop_top input; moveDown output; moveUp output
  data driver_neutral settings: description=$TL$ type=Bool; $TL$
  data driver_up settings: description=$TL$ type=Bool; $TL$
  data driver_down settings: description=$TL$ type=Bool; $TL$
  data passenger_neutral settings: description=$TL$ type=Bool; $TL$
  data passenger_up settings: description=$TL$ type=Bool; $TL$
  data passenger_down settings: description=$TL$ type=Bool; $TL$
  data obstacle settings: description=$TL$ type=Bool; $TL$
  data endstop_bottom settings: description=$TL$ type=Bool; $TL$
  data endstop_top settings: description=$TL$ type=Bool; $TL$
